simulink library "lib_electric_machine"  (Simulink 4.1.1)
undefined symbols (not defined in the file or in its folder): amb_tmp, cyc_mph, ess_module_num, ess_voc, fd_ratio, gb_num_init, gb_ratio, gc_cp, gc_inertia, gc_inpwr_map, gc_map_spd, gc_map_trq, gc_mass, gc_max_crrnt, gc_max_trq, gc_outpwr_map, gc_overtrq_factor, gc_sarea, gc_spd_scale, gc_th_calc, gc_trq_scale, gc_tstat, mc_cp, mc_eff_scale, mc_inertia, mc_init_tmp, mc_inpwr_map, mc_map_spd, mc_map_trq, mc_mass, mc_max_gen_trq, mc_max_trq, mc_overtrq_factor, mc_sarea, mc_spd_scale, mc_th_calc, mc_trq_scale, mc_tstat, tc_mc_to_fc_ratio, veh_mass, wh_radius
libraries: lib_electric_machine x4
(part 2 of 2)

== system lib_electric_machine/motor/ controller <mc> prius/N-m drive torque per W input ==
  req'd input power (W) : Inport  Port=1  LatchInput=off
  req'd rotor drive torque (Nm) : Inport  Port=2  LatchInput=off
  Block NOTES : Subsystem
      settings: RTWFcnNameOpts=Auto  RTWFileNameOpts=Auto
      mask Display: disp('Block\nNOTES')
  Constant : Constant  Value=eps
  Constant1 : Constant  Value=0
  Constant2 : Constant  Value=inf
  Product : Product  Inputs=/*  Multiplication=Element-wise(.*)  SaturateOnIntegerOverflow=on
  Relational Operator : RelationalOperator  Operator=~=
  Sum : Sum  Inputs=++  SaturateOnIntegerOverflow=on
  Switch : Switch  Threshold=eps
  Nm per W : Outport  Port=1  InitialOutput=0
  wires:
  Constant/1 -> Sum/1
  req'd rotor drive torque (Nm)/1 -> Product/2
  Product/1 -> Switch/1
  Relational Operator/1 -> Switch/2
  Switch/1 -> Nm per W/1
  Sum/1 -> Product/1
  req'd input power (W)/1 -> Sum/2, Relational Operator/1
  Constant1/1 -> Relational Operator/2
  Constant2/1 -> Switch/3

== system lib_electric_machine/motor/ controller <mc> prius/documentation10 ==

== system lib_electric_machine/motor/ controller <mc> prius/effect of inertia (Nm) ==
  mc_spd_out_a : Inport  Port=1  LatchInput=off
  Block NOTES : Subsystem
      settings: RTWFcnNameOpts=Auto  RTWFileNameOpts=Auto
      mask Display: disp('Block\nNOTES')
  Constant : Constant  Value=eps
  Constant1 : Constant  Value=max(mc_max_trq)*mc_trq_scale*mc_overtrq_factor
  Constant2 : Constant  Orientation=left  Value=fd_ratio/wh_radius
  Gain : Gain  Gain=mc_inertia  Multiplication=Element-wise(K.*u)  SaturateOnIntegerOverflow=on
  Memory : Memory  X0=0  InheritSampleTime=off
      settings: RTWStateStorageClass=Auto
  MinMax : MinMax  Function=min  Inputs=2
  Product : Product  Inputs=2  Multiplication=Element-wise(.*)  SaturateOnIntegerOverflow=on
  Sum : Sum  Inputs=++  SaturateOnIntegerOverflow=on
  Switch : Switch  Threshold=eps
  alpha : Derivative
  motor inertia as a function of total vehicle inertia (generous approximation) : lib_electric_machine/Sub-models/motor inertia as a function of total vehicle inertia (generous approximation)  Orientation=up
  overall gear ratio / wh_radius : Product  Inputs=*/  Multiplication=Element-wise(.*)  SaturateOnIntegerOverflow=on
  out_1 : Outport  Port=1  InitialOutput=0
  wires:
  alpha/1 -> Gain/1
  mc_spd_out_a/1 -> alpha/1, overall gear ratio / wh_radius/1
  MinMax/1 -> out_1/1
  Gain/1 -> MinMax/1
  Product/1 -> MinMax/2
  overall gear ratio / wh_radius/1 -> Memory/1
  Constant1/1 -> Product/1
  Memory/1 -> motor inertia as a function of total vehicle inertia (generous approximation)/1
  motor inertia as a function of total vehicle inertia (generous approximation)/1 -> Product/2
  Constant/1 -> Sum/2
  Sum/1 -> Switch/1
  [veh_spd_a_rec] -> Sum/1, Switch/2
  Constant2/1 -> Switch/3
  Switch/1 -> overall gear ratio / wh_radius/2

== system lib_electric_machine/motor/ controller <mc> prius/enforce torque limit ==
  req'd motor torque (Nm) : Inport  Port=1  LatchInput=off
  limited motor speed (rad/s) : Inport  Port=2  LatchInput=off
  Block NOTES : Subsystem
      settings: RTWFcnNameOpts=Auto  RTWFileNameOpts=Auto
      mask Display: disp('Block\nNOTES')
  MinMax : MinMax  Function=min  Inputs=2
  MinMax1 : MinMax  Function=max  Inputs=2
  Relational Operator2 : RelationalOperator  Operator=~=
  Switch : Switch  Threshold=0
  To WS2 : ToWorkspace  VariableName=mc_max_trq_vec  SampleTime=0  SaveFormat=Array
      settings: MaxDataPoints=50000
  max gen torque : Lookup  InputValues=mc_map_spd*mc_spd_scale  OutputValues=mc_max_gen_trq*mc_overtrq_factor*mc_trq_scale
  max torque : Lookup  InputValues=mc_map_spd*mc_spd_scale  OutputValues=mc_max_trq*mc_overtrq_factor*mc_trq_scale
  limited motor torque (Nm) : Outport  Port=1
  tag scope: mc_trq_limited=global
  wires:
  max torque/1 -> To WS2/1, MinMax/2
  req'd motor torque (Nm)/1 -> Relational Operator2/1, Switch/2, MinMax1/1, MinMax/1
  Switch/1 -> Relational Operator2/2, limited motor torque (Nm)/1
  MinMax1/1 -> Switch/3
  MinMax/1 -> Switch/1
  Relational Operator2/1 -> [mc_trq_limited]
  limited motor speed (rad/s)/1 -> max torque/1, max gen torque/1
  max gen torque/1 -> MinMax1/2

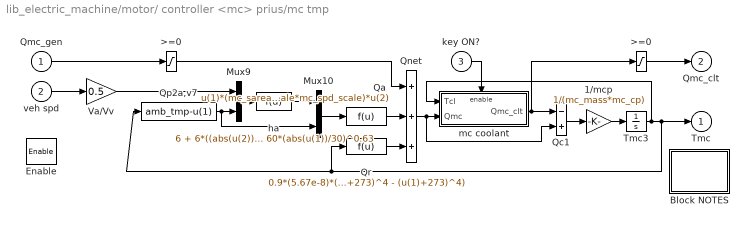
== system lib_electric_machine/motor/ controller <mc> prius/mc tmp ==
  Qmc_gen : Inport  Port=1  LatchInput=off
  veh spd : Inport  Port=2  LatchInput=off
  key ON? : Inport  Port=3  LatchInput=off
  Enable : EnablePort  StatesWhenEnabling=reset
  1/mcp : Gain  Gain=1/(mc_mass*mc_cp)  Multiplication=Element-wise(K.*u)  SaturateOnIntegerOverflow=on
  >=0 : Saturate  UpperLimit=Inf  LowerLimit=0  LinearizeAsGain=on
  ">=0 " : Saturate  UpperLimit=Inf  LowerLimit=0  LinearizeAsGain=on
  Block NOTES : Subsystem
      settings: RTWFcnNameOpts=Auto  RTWFileNameOpts=Auto
      mask Display: disp('Block\nNOTES')
  Mux10 : Mux  Inputs=2
      settings: DisplayOption=none
  Mux9 : Mux  Inputs=2
      settings: DisplayOption=none
  Qa : Fcn  Expr=u(1)*(mc_sarea*mc_trq_scale*mc_spd_scale)*u(2)
  Qc1 : Sum  Inputs=-+  SaturateOnIntegerOverflow=on
  Qnet : Sum  Inputs=+++  SaturateOnIntegerOverflow=on
  Qp2a,v7 : Fcn  Expr=amb_tmp-u(1)
  Qr : Fcn  Expr=0.9*(5.67e-8)*(mc_sarea*mc_trq_scale*mc_spd_scale)*((amb_tmp+273)^4 - (u(1)+273)^4)
  Tmc3 : Integrator  ExternalReset=none  InitialConditionSource=internal  InitialCondition=mc_init_tmp  LimitOutput=off  UpperSaturationLimit=inf  LowerSaturationLimit=-inf  ShowSaturationPort=off  ShowStatePort=off  AbsoluteTolerance=auto
  Va/Vv : Gain  Gain=0.5  Multiplication=Element-wise(K.*u)  SaturateOnIntegerOverflow=on
  ha : Fcn  Expr=6 + 6*((abs(u(2))/1000))^0.25 + 60*(abs(u(1))/30)^0.63
  mc coolant : Subsystem  TreatAsAtomicUnit=on
      settings: RTWFcnNameOpts=Auto  RTWFileNameOpts=Auto
  Tmc : Outport  Port=1  InitialOutput=0
  Qmc_clt : Outport  Port=2  OutputWhenDisabled=reset  InitialOutput=0
  wires:
  Mux10/1 -> Qa/1
  Mux9/1 -> ha/1
  Va/Vv/1 -> Mux9/1
  ha/1 -> Mux10/1
  Qp2a,v7/1 -> Mux9/2, Mux10/2
  Qr/1 -> Qnet/3
  Qmc_gen/1 -> ">=0 "/1
  ">=0 "/1 -> Qnet/1
  Qa/1 -> Qnet/2
  veh spd/1 -> Va/Vv/1
  key ON?/1 -> mc coolant/Enable
  >=0/1 -> Qmc_clt/1
  mc coolant/1(Qmc_clt) -> >=0/1, Qc1/1
  Tmc3/1 -> mc coolant/1(Tcl), Tmc/1, Qr/1, Qp2a,v7/1
  1/mcp/1 -> Tmc3/1
  Qc1/1 -> 1/mcp/1
  Qnet/1 -> mc coolant/2("Qmc "), Qc1/2

== system lib_electric_machine/motor/ controller <mc> prius/motor controller logic interface ==
  w_mc_out_r : Inport  Port=1  LatchInput=off
  P_mc_in_1lim : Inport  Port=2  LatchInput=off
  P_mc_in_r : Outport  Port=1  InitialOutput=0
  tag scope: P_mc_in_1lim=global, w_mc_out_r=global
  wires:
  P_mc_in_1lim/1 -> [P_mc_in_1lim]
  w_mc_out_r/1 -> [w_mc_out_r]
  [P_mc_in_r] -> P_mc_in_r/1

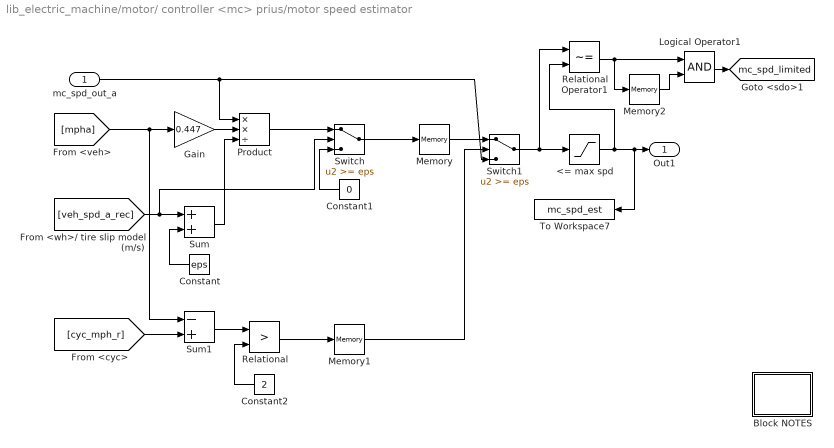
== system lib_electric_machine/motor/ controller <mc> prius/motor speed estimator ==
  mc_spd_out_a : Inport  Port=1  LatchInput=off
  <= max spd : Saturate  UpperLimit=max(mc_map_spd)*mc_spd_scale  LowerLimit=-inf  LinearizeAsGain=on
  Block NOTES : Subsystem
      settings: RTWFcnNameOpts=Auto  RTWFileNameOpts=Auto
      mask Display: disp('Block\nNOTES')
  Constant : Constant  Orientation=left  Value=eps
  Constant1 : Constant  Orientation=left  Value=0
  Constant2 : Constant  Orientation=left  Value=2
  Gain : Gain  Gain=0.447  Multiplication=Element-wise(K.*u)  SaturateOnIntegerOverflow=on
  Logical Operator1 : Logic  Operator=AND  Inputs=2
  Memory : Memory  X0=cyc_mph(1,2)*0.447/wh_radius*fd_ratio  InheritSampleTime=off
      settings: RTWStateStorageClass=Auto
  Memory1 : Memory  X0=1  InheritSampleTime=off
      settings: RTWStateStorageClass=Auto
  Memory2 : Memory  X0=0  InheritSampleTime=off
      settings: RTWStateStorageClass=Auto
  Product : Product  Inputs=**/  Multiplication=Element-wise(.*)  SaturateOnIntegerOverflow=on
  Relational : RelationalOperator  Operator=>
  Relational Operator1 : RelationalOperator  Operator=~=
  Sum : Sum  Inputs=++  SaturateOnIntegerOverflow=on
  Sum1 : Sum  Inputs=-+  SaturateOnIntegerOverflow=on
  Switch : Switch  Threshold=eps
  Switch1 : Switch  Threshold=eps
  To Workspace7 : ToWorkspace  VariableName=mc_spd_est  SampleTime=-1  SaveFormat=Array
  Out1 : Outport  Port=1
  tag scope: mc_spd_limited=global
  wires:
  <= max spd/1 -> Relational Operator1/2, To Workspace7/1, Out1/1
  Switch1/1 -> Relational Operator1/1, <= max spd/1
  Relational Operator1/1 -> Memory2/1, Logical Operator1/1
  Logical Operator1/1 -> [mc_spd_limited]
  Memory2/1 -> Logical Operator1/2
  mc_spd_out_a/1 -> Switch1/3, Product/1
  Product/1 -> Switch/1
  Sum/1 -> Product/3
  Gain/1 -> Product/2
  [veh_spd_a_rec] -> Sum/1, Switch/2
  Constant1/1 -> Switch/3
  Memory/1 -> Switch1/1
  Constant/1 -> Sum/2
  [cyc_mph_r] -> Sum1/2
  [mpha] -> Gain/1, Sum1/1
  Constant2/1 -> Relational/2
  Sum1/1 -> Relational/1
  Relational/1 -> Memory1/1
  Memory1/1 -> Switch1/2
  Switch/1 -> Memory/1

== system lib_electric_machine/motor/ controller <mc> prius/rotor drive torque available (Nm) ==
  torque per unit input power (N-m/W) : Inport  Port=1  LatchInput=off
  available input power (W) : Inport  Port=2  LatchInput=off
  Block NOTES : Subsystem
      settings: RTWFcnNameOpts=Auto  RTWFileNameOpts=Auto
      mask Display: disp('Block\nNOTES')
  Constant2 : Constant  Value=inf
  Constant3 : Constant  Value=0
  Product : Product  Inputs=2  Multiplication=Element-wise(.*)  SaturateOnIntegerOverflow=on
  Relational Operator : RelationalOperator  Operator=~=
  Switch : Switch  Threshold=eps
  rotor drive torque available : Outport  Port=1  InitialOutput=0
  wires:
  torque per unit input power (N-m/W)/1 -> Relational Operator/1, Product/1
  Switch/1 -> rotor drive torque available/1
  Relational Operator/1 -> Switch/2
  Product/1 -> Switch/1
  available input power (W)/1 -> Product/2
  Constant2/1 -> Relational Operator/2
  Constant3/1 -> Switch/3

== system lib_electric_machine/prius gen/ controller <gc>/Block NOTES ==
  note: This generator/controller model includes loss data, rotational inertia, and performance limits.
  note: Available torque is computed from available power by assuming that the ratio of rotor torque to input
      | (electric) power is the same for the actual/achievable situation as was computed for the request.  This
      | is mathematically equivalent to assuming that the generator/controller efficiency.  Rotor speed for the
      | actual/achievable calculations is as computed in the 'request' branch.

== system lib_electric_machine/prius gen/ controller <gc>/N-m drive torque per W input ==
  req'd input power (W) : Inport  Port=1  LatchInput=off
  req'd rotor drive torque (Nm) : Inport  Port=2  LatchInput=off
  Block NOTES : Subsystem
      settings: RTWFcnNameOpts=Auto  RTWFileNameOpts=Auto
      mask Display: disp('Block\nNOTES')
  Constant : Constant  Value=eps
  Constant1 : Constant  Value=0
  Constant2 : Constant  Value=inf
  Product : Product  Inputs=/*  Multiplication=Element-wise(.*)  SaturateOnIntegerOverflow=on
  Relational Operator : RelationalOperator  Operator=~=
  Sum : Sum  Inputs=++  SaturateOnIntegerOverflow=on
  Switch : Switch  Threshold=eps
  Nm per W : Outport  Port=1  InitialOutput=0
  wires:
  Constant/1 -> Sum/1
  req'd rotor drive torque (Nm)/1 -> Product/2
  Product/1 -> Switch/1
  Relational Operator/1 -> Switch/2
  Switch/1 -> Nm per W/1
  Sum/1 -> Product/1
  req'd input power (W)/1 -> Sum/2, Relational Operator/1
  Constant1/1 -> Relational Operator/2
  Constant2/1 -> Switch/3

== system lib_electric_machine/prius gen/ controller <gc>/effect of inertia (Nm) ==
  in_1 : Inport  Port=1  LatchInput=off
  Gain : Gain  Gain=gc_inertia  Multiplication=Element-wise(K.*u)  SaturateOnIntegerOverflow=on
  To Workspace9 : ToWorkspace  VariableName=gc_inertia_trq  SampleTime=-1  SaveFormat=Array
      settings: Orientation=up
  alpha : Derivative
  out_1 : Outport  Port=1  InitialOutput=0
  wires:
  in_1/1 -> alpha/1
  alpha/1 -> Gain/1
  Gain/1 -> out_1/1, To Workspace9/1

== system lib_electric_machine/prius gen/ controller <gc>/enforce torque limit ==
  req'd gen torque (Nm) : Inport  Port=1  LatchInput=off
  limited gen speed (rad/s) : Inport  Port=2  LatchInput=off
  Block NOTES : Subsystem
      settings: RTWFcnNameOpts=Auto  RTWFileNameOpts=Auto
      mask Display: disp('Block\nNOTES')
  Gain : Gain  Gain=-1  Multiplication=Element-wise(K.*u)  SaturateOnIntegerOverflow=on
  MinMax : MinMax  Function=min  Inputs=2
  MinMax1 : MinMax  Function=max  Inputs=2
  Relational Operator2 : RelationalOperator  Operator=~=
  Switch : Switch  Threshold=0
  max torque : Lookup  InputValues=gc_map_spd*gc_spd_scale  OutputValues=gc_max_trq*gc_overtrq_factor*gc_trq_scale
  limited generator torque (Nm) : Outport  Port=1
  tag scope: gc_trq_limited=global
  wires:
  Relational Operator2/1 -> [gc_trq_limited]
  max torque/1 -> MinMax/2, Gain/1
  MinMax/1 -> Switch/1
  MinMax1/1 -> Switch/3
  Gain/1 -> MinMax1/2
  limited gen speed (rad/s)/1 -> max torque/1
  Switch/1 -> limited generator torque (Nm)/1, Relational Operator2/2
  req'd gen torque (Nm)/1 -> MinMax/1, MinMax1/1, Switch/2, Relational Operator2/1

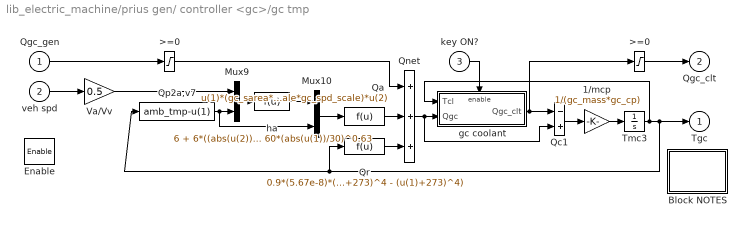
== system lib_electric_machine/prius gen/ controller <gc>/gc tmp ==
  Qgc_gen : Inport  Port=1  LatchInput=off
  veh spd : Inport  Port=2  LatchInput=off
  key ON? : Inport  Port=3  LatchInput=off
  Enable : EnablePort  StatesWhenEnabling=reset
  1/mcp : Gain  Gain=1/(gc_mass*gc_cp)  Multiplication=Element-wise(K.*u)  SaturateOnIntegerOverflow=on
  >=0 : Saturate  UpperLimit=Inf  LowerLimit=0  LinearizeAsGain=on
  ">=0 " : Saturate  UpperLimit=Inf  LowerLimit=0  LinearizeAsGain=on
  Block NOTES : Subsystem
      settings: RTWFcnNameOpts=Auto  RTWFileNameOpts=Auto
      mask Display: disp('Block\nNOTES')
  Mux10 : Mux  Inputs=2
      settings: DisplayOption=none
  Mux9 : Mux  Inputs=2
      settings: DisplayOption=none
  Qa : Fcn  Expr=u(1)*(gc_sarea*gc_trq_scale*gc_spd_scale)*u(2)
  Qc1 : Sum  Inputs=-+  SaturateOnIntegerOverflow=on
  Qnet : Sum  Inputs=+++  SaturateOnIntegerOverflow=on
  Qp2a,v7 : Fcn  Expr=amb_tmp-u(1)
  Qr : Fcn  Expr=0.9*(5.67e-8)*(mc_sarea*mc_trq_scale*gc_spd_scale)*((amb_tmp+273)^4 - (u(1)+273)^4)
  Tmc3 : Integrator  ExternalReset=none  InitialConditionSource=internal  InitialCondition=mc_init_tmp  LimitOutput=off  UpperSaturationLimit=inf  LowerSaturationLimit=-inf  ShowSaturationPort=off  ShowStatePort=off  AbsoluteTolerance=auto
  Va/Vv : Gain  Gain=0.5  Multiplication=Element-wise(K.*u)  SaturateOnIntegerOverflow=on
  gc coolant : Subsystem  TreatAsAtomicUnit=on
      settings: RTWFcnNameOpts=Auto  RTWFileNameOpts=Auto
  ha : Fcn  Expr=6 + 6*((abs(u(2))/1000))^0.25 + 60*(abs(u(1))/30)^0.63
  Tgc : Outport  Port=1  InitialOutput=0
  Qgc_clt : Outport  Port=2  OutputWhenDisabled=reset  InitialOutput=0
  wires:
  Qnet/1 -> Qc1/2, gc coolant/2("Qgc ")
  Qc1/1 -> 1/mcp/1
  1/mcp/1 -> Tmc3/1
  Tmc3/1 -> Qp2a,v7/1, Qr/1, Tgc/1, gc coolant/1(Tcl)
  gc coolant/1(Qgc_clt) -> Qc1/1, >=0/1
  >=0/1 -> Qgc_clt/1
  key ON?/1 -> gc coolant/Enable
  veh spd/1 -> Va/Vv/1
  Qa/1 -> Qnet/2
  ">=0 "/1 -> Qnet/1
  Qgc_gen/1 -> ">=0 "/1
  Qr/1 -> Qnet/3
  Qp2a,v7/1 -> Mux10/2, Mux9/2
  ha/1 -> Mux10/1
  Va/Vv/1 -> Mux9/1
  Mux9/1 -> ha/1
  Mux10/1 -> Qa/1

== system lib_electric_machine/prius gen/ controller <gc>/gen controller logic interface ==
  w_gc_out_r : Inport  Port=1  LatchInput=off
  P_gc_in_1lim : Inport  Port=2  LatchInput=off
  P_gc_in_r : Outport  Port=1  InitialOutput=0
  tag scope: P_gc_in_1lim=global, w_gc_out_r=global
  wires:
  P_gc_in_1lim/1 -> [P_gc_in_1lim]
  w_gc_out_r/1 -> [w_gc_out_r]
  [P_gc_in_r] -> P_gc_in_r/1

== system lib_electric_machine/prius gen/ controller <gc>/rotor drive torque available (Nm) ==
  torque per unit input power (N-m/W) : Inport  Port=1  LatchInput=off
  available input power (W) : Inport  Port=2  LatchInput=off
  Block NOTES : Subsystem
      settings: RTWFcnNameOpts=Auto  RTWFileNameOpts=Auto
      mask Display: disp('Block\nNOTES')
  Constant2 : Constant  Value=inf
  Constant3 : Constant  Value=0
  Product : Product  Inputs=2  Multiplication=Element-wise(.*)  SaturateOnIntegerOverflow=on
  Relational Operator : RelationalOperator  Operator=~=
  Switch : Switch  Threshold=eps
  rotor drive torque available : Outport  Port=1  InitialOutput=0
  wires:
  torque per unit input power (N-m/W)/1 -> Relational Operator/1, Product/1
  Switch/1 -> rotor drive torque available/1
  Relational Operator/1 -> Switch/2
  Product/1 -> Switch/1
  available input power (W)/1 -> Product/2
  Constant2/1 -> Relational Operator/2
  Constant3/1 -> Switch/3

== system lib_electric_machine/generator/ controller <gc>/enforce torque limit/Block NOTES ==
  note: This block enforces the maximum torque
      | absorption capability limit of the generator.

== system lib_electric_machine/generator/ controller <gc>/limit request: controller current limit/Block NOTES ==
  note: This block prevents the generator/controller set from
      | outputting more than its maximum rated current.

== system lib_electric_machine/motor/ controller <mc>/N-m drive torque per W input/Block NOTES ==
  note: This block determines the ratio of req'd rotor torque to req'd electrical input power,
      |  which is proportional to efficiency if the motor is providing torque.  This ratio is used
      | to compute actual rotor torque given some input power which may be different from
      | the req'd value.
      |
      | If the denominator, the req'd input power, is zero, this block outputs inf,
      | which is a flag used by the block .../rotor drive torque available (Nm).

== system lib_electric_machine/motor/ controller <mc>/effect of inertia (Nm)/Block NOTES ==
  note: Torque required to accelerate the motor's inertia is calculated from the rate of change
      | of mc_spd_out_a.  It is no greater than the product of the maximum motor torque and
      | the fractional contribution of the motor's inertia to the total vehicle inertia.

== system lib_electric_machine/motor/ controller <mc>/enforce torque limit/Block NOTES ==
  note: This block enforces the maximum torque production and absorption
      | capability limits of the motor.  It assumes that exactly as much torque
      | can be absorbed as can be produced at a given speed.

== system lib_electric_machine/motor/ controller <mc>/mc tmp/Block NOTES ==
  note: This block models the thermal behavior of a motor
      | and controller  with active fluid cooling.
      | The module is modeled as a single lumped thermal mass.
      | The fan is on whenever the battery temp is > the set temp.

== system lib_electric_machine/motor/ controller <mc>/mc tmp/mc coolant ==
  Tcl : Inport  Port=1  LatchInput=off
  "Qmc " : Inport  Port=2  LatchInput=off
  Enable : EnablePort  StatesWhenEnabling=reset
  Constant : Constant  Value=mc_tstat
  Product1 : Product  Inputs=2  Multiplication=Element-wise(.*)  SaturateOnIntegerOverflow=on
  Relational Operator : RelationalOperator  Operator=<=
  Qmc_clt : Outport  Port=1  OutputWhenDisabled=reset  InitialOutput=0
  wires:
  Relational Operator/1 -> Product1/1
  Product1/1 -> Qmc_clt/1
  "Qmc "/1 -> Product1/2
  Constant/1 -> Relational Operator/1
  Tcl/1 -> Relational Operator/2

== system lib_electric_machine/motor/ controller <mc>/motor speed estimator/Block NOTES ==
  note: The requested motor speed is replaced by an estimate of the
      | motor's previous speed, for loss and max. torque calculations,
      | whenever the vehicle missed the trace by more than 1 mph
      | on the last time step.

== system lib_electric_machine/motor/ controller <mc>/rotor drive torque available (Nm)/Block NOTES ==
  note: This block computes the actual rotor torque given the actual motor input power and
      | the ratio (req'd rotor torque)/(req'd input power).
      |
      | If the above ratio has the value inf, which implies that the req'd input power is zero,
      | then the actual rotor torque is assumed to be zero.  This is not reflective of reality, of course:
      | with zero input power, the rotor torque would be the motor spin-loss torque at the given speed.
      | Because this simplification occurs only when req'd input power is zero, it does not.
      | affect fuel economy or max effort acceleration calculations.

== system lib_electric_machine/motor/ controller <mc> par/N-m drive torque per W input/Block NOTES ==
  note: This block determines the ratio of req'd rotor torque to req'd electrical input power,
      |  which is proportional to efficiency if the motor is providing torque.  This ratio is used
      | to compute actual rotor torque given some input power which may be different from
      | the req'd value.
      |
      | If the denominator, the req'd input power, is zero, this block outputs inf,
      | which is a flag used by the block .../rotor drive torque available (Nm).

== system lib_electric_machine/motor/ controller <mc> par/effect of inertia (Nm)/Block NOTES ==
  note: Torque required to accelerate the motor's inertia is calculated from the rate of change
      | of mc_spd_out_a.  It is no greater than the product of the maximum motor torque and
      | the fractional contribution of the motor's inertia to the total vehicle inertia.

== system lib_electric_machine/motor/ controller <mc> par/enforce torque limit/Block NOTES ==
  note: This block enforces the maximum torque production and absorption
      | capability limits of the motor.  It assumes that exactly as much torque
      | can be absorbed as can be produced at a given speed.

== system lib_electric_machine/motor/ controller <mc> par/mc tmp/Block NOTES ==
  note: This block models the thermal behavior of a motor
      | and controller  with active fluid cooling.
      | The module is modeled as a single lumped thermal mass.
      | The fan is on whenever the battery temp is > the set temp.

== system lib_electric_machine/motor/ controller <mc> par/mc tmp/mc coolant ==
  Tcl : Inport  Port=1  LatchInput=off
  "Qmc " : Inport  Port=2  LatchInput=off
  Enable : EnablePort  StatesWhenEnabling=reset
  Constant : Constant  Value=mc_tstat
  Product1 : Product  Inputs=2  Multiplication=Element-wise(.*)  SaturateOnIntegerOverflow=on
  Relational Operator : RelationalOperator  Operator=<=
  Qmc_clt : Outport  Port=1  OutputWhenDisabled=reset  InitialOutput=0
  wires:
  Relational Operator/1 -> Product1/1
  Product1/1 -> Qmc_clt/1
  "Qmc "/1 -> Product1/2
  Constant/1 -> Relational Operator/1
  Tcl/1 -> Relational Operator/2

== system lib_electric_machine/motor/ controller <mc> par/motor speed estimator/Block NOTES ==
  note: The requested motor speed is replaced by an estimate of the
      | motor's previous speed, for loss and max. torque calculations,
      | whenever the vehicle missed the trace by more than 1 mph
      | on the last time step.

== system lib_electric_machine/motor/ controller <mc> par/rotor drive torque available (Nm)/Block NOTES ==
  note: This block computes the actual rotor torque given the actual motor input power and
      | the ratio (req'd rotor torque)/(req'd input power).
      |
      | If the above ratio has the value inf, which implies that the req'd input power is zero,
      | then the actual rotor torque is assumed to be zero.  This is not reflective of reality, of course:
      | with zero input power, the rotor torque would be the motor spin-loss torque at the given speed.
      | Because this simplification occurs only when req'd input power is zero, it does not.
      | affect fuel economy or max effort acceleration calculations.

== system lib_electric_machine/motor/ controller <mc> prius/N-m drive torque per W input/Block NOTES ==
  note: This block determines the ratio of req'd rotor torque to req'd electrical input power,
      |  which is proportional to efficiency if the motor is providing torque.  This ratio is used
      | to compute actual rotor torque given some input power which may be different from
      | the req'd value.
      |
      | If the denominator, the req'd input power, is zero, this block outputs inf,
      | which is a flag used by the block .../rotor drive torque available (Nm).

== system lib_electric_machine/motor/ controller <mc> prius/effect of inertia (Nm)/Block NOTES ==
  note: Torque required to accelerate the motor's inertia is calculated from the rate of change
      | of mc_spd_out_a.  It is no greater than the product of the maximum motor torque and
      | the fractional contribution of the motor's inertia to the total vehicle inertia.

== system lib_electric_machine/motor/ controller <mc> prius/enforce torque limit/Block NOTES ==
  note: This block enforces the maximum torque production and absorption
      | capability limits of the motor.  It assumes that exactly as much torque
      | can be absorbed as can be produced at a given speed.

== system lib_electric_machine/motor/ controller <mc> prius/mc tmp/Block NOTES ==
  note: This block models the thermal behavior of a motor
      | and controller  with active fluid cooling.
      | The module is modeled as a single lumped thermal mass.
      | The fan is on whenever the battery temp is > the set temp.

== system lib_electric_machine/motor/ controller <mc> prius/mc tmp/mc coolant ==
  Tcl : Inport  Port=1  LatchInput=off
  "Qmc " : Inport  Port=2  LatchInput=off
  Enable : EnablePort  StatesWhenEnabling=reset
  Constant : Constant  Value=mc_tstat
  Product1 : Product  Inputs=2  Multiplication=Element-wise(.*)  SaturateOnIntegerOverflow=on
  Relational Operator : RelationalOperator  Operator=<=
  Qmc_clt : Outport  Port=1  OutputWhenDisabled=reset  InitialOutput=0
  wires:
  Relational Operator/1 -> Product1/1
  Product1/1 -> Qmc_clt/1
  "Qmc "/1 -> Product1/2
  Constant/1 -> Relational Operator/1
  Tcl/1 -> Relational Operator/2

== system lib_electric_machine/motor/ controller <mc> prius/motor speed estimator/Block NOTES ==
  note: The requested motor speed is replaced by an estimate of the
      | motor's previous speed, for loss and max. torque calculations,
      | whenever the vehicle missed the trace by more than 1 mph
      | on the last time step.

== system lib_electric_machine/motor/ controller <mc> prius/rotor drive torque available (Nm)/Block NOTES ==
  note: This block computes the actual rotor torque given the actual motor input power and
      | the ratio (req'd rotor torque)/(req'd input power).
      |
      | If the above ratio has the value inf, which implies that the req'd input power is zero,
      | then the actual rotor torque is assumed to be zero.  This is not reflective of reality, of course:
      | with zero input power, the rotor torque would be the motor spin-loss torque at the given speed.
      | Because this simplification occurs only when req'd input power is zero, it does not.
      | affect fuel economy or max effort acceleration calculations.

== system lib_electric_machine/prius gen/ controller <gc>/N-m drive torque per W input/Block NOTES ==
  note: This block determines the ratio of req'd rotor torque to req'd electrical input power,
      |  which is proportional to efficiency if the motor is providing torque.  This ratio is used
      | to compute actual rotor torque given some input power which may be different from
      | the req'd value.
      |
      | If the denominator, the req'd input power, is zero, this block outputs inf,
      | which is a flag used by the block .../rotor drive torque available (Nm).

== system lib_electric_machine/prius gen/ controller <gc>/enforce torque limit/Block NOTES ==
  note: This block enforces the maximum torque production and absorption
      | capability limits of the generator.  It assumes that exactly as much torque
      | can be absorbed as can be produced at a given speed.

== system lib_electric_machine/prius gen/ controller <gc>/gc tmp/Block NOTES ==
  note: This block models the thermal behavior of a motor/generator
      | and controller  with active fluid cooling.
      | The module is modeled as a single lumped thermal mass.
      | The fan is on whenever the battery temp is > the set temp.

== system lib_electric_machine/prius gen/ controller <gc>/gc tmp/gc coolant ==
  Tcl : Inport  Port=1  LatchInput=off
  "Qgc " : Inport  Port=2  LatchInput=off
  Enable : EnablePort  StatesWhenEnabling=reset
  Constant : Constant  Value=gc_tstat
  Product1 : Product  Inputs=2  Multiplication=Element-wise(.*)  SaturateOnIntegerOverflow=on
  Relational Operator : RelationalOperator  Operator=<=
  Qgc_clt : Outport  Port=1  OutputWhenDisabled=reset  InitialOutput=0
  wires:
  Tcl/1 -> Relational Operator/2
  Constant/1 -> Relational Operator/1
  "Qgc "/1 -> Product1/2
  Product1/1 -> Qgc_clt/1
  Relational Operator/1 -> Product1/1

== system lib_electric_machine/prius gen/ controller <gc>/rotor drive torque available (Nm)/Block NOTES ==
  note: This block computes the actual rotor torque given the actual motor input power and
      | the ratio (req'd rotor torque)/(req'd input power).
      |
      | If the above ratio has the value inf, which implies that the req'd input power is zero,
      | then the actual rotor torque is assumed to be zero.  This is not reflective of reality, of course:
      | with zero input power, the rotor torque would be the motor spin-loss torque at the given speed.
      | Because this simplification occurs only when req'd input power is zero, it does not.
      | affect fuel economy or max effort acceleration calculations.
